simulink model "modeloSatDead"  (R2024b)
settings: Solver=VariableStepAuto  StartTime=0.0  StopTime=10  RelTol=1e-3
undefined symbols (not defined in the file): step_value
settings Model: Creator=estel  LastModifiedBy=estel

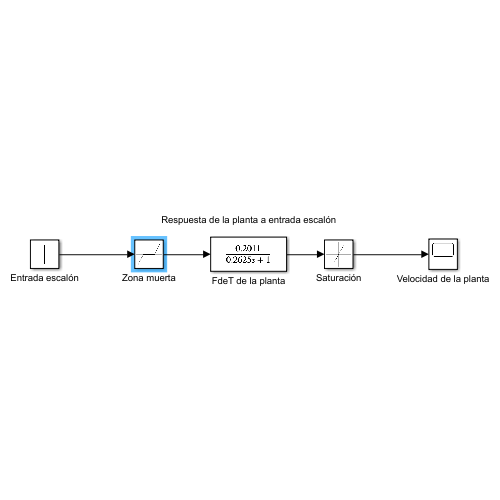
[thumbnail: Simulink's stored preview of the top-level diagram]
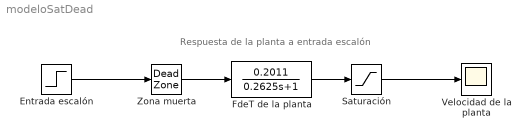
== system modeloSatDead ==
  note: Respuesta de la planta a entrada escalón
  Entrada escalón : Step  Time=0  After=step_value  SampleTime=0
  FdeT de la planta : TransferFcn  Numerator=0.2011  Denominator=[0.2625 1]
  Saturación : Saturate  UpperLimit=2.1098  LowerLimit=-2.1123
  Velocidad de la planta : Scope
  Zona muerta : DeadZone  LowerValue=-0.20  UpperValue=0.21
  wires:
  Entrada escalón/1 -> Zona muerta/1
  Saturación/1 -> Velocidad de la planta/1
  FdeT de la planta/1 -> Saturación/1
  Zona muerta/1 -> FdeT de la planta/1
